simulink subsystem "PieroHFModel"  (R2023b)
settings: Solver=VariableStepAuto  StartTime=0.0  StopTime=10.0  RelTol=1e-3
settings Model: Creator=Hajar  LastModifiedBy=Hajar

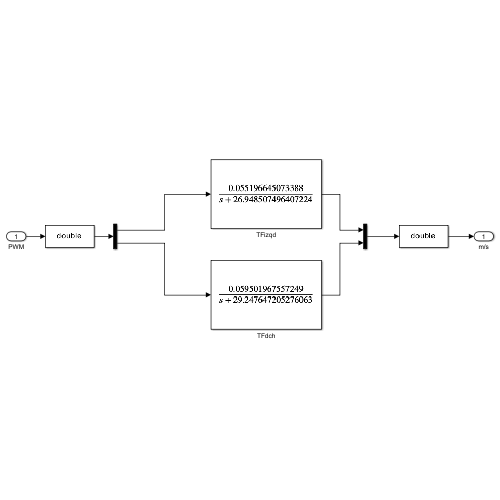
[thumbnail: Simulink's stored preview of the top-level diagram]
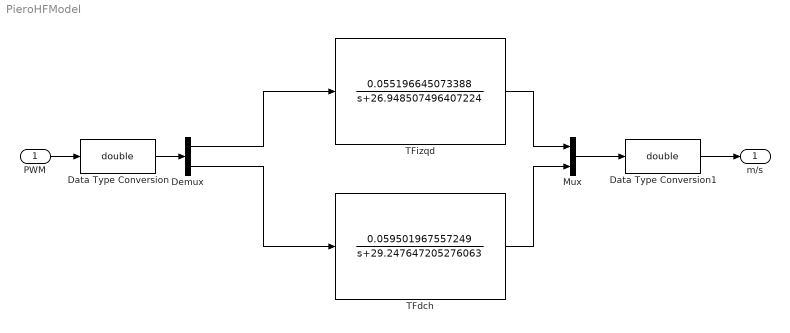
== system PieroHFModel ==
  PWM : Inport
  Data Type Conversion : DataTypeConversion  OutDataTypeStr=double  SaturateOnIntegerOverflow=off  RndMeth=Floor
  Data Type Conversion1 : DataTypeConversion  OutDataTypeStr=double  SaturateOnIntegerOverflow=off  RndMeth=Floor
  Demux : Demux  Outputs=2
  Mux : Mux  Inputs=2
  TFdch : TransferFcn  Numerator=0.059501967557249  Denominator=[1,29.247647205276063]
  TFizqd : TransferFcn  Numerator=0.055196645073388  Denominator=[1,26.948507496407224]
  m/s : Outport
  wires:
  Demux/1 -> TFizqd/1
  Demux/2 -> TFdch/1
  TFizqd/1 -> Mux/1
  TFdch/1 -> Mux/2
  PWM/1 -> Data Type Conversion/1
  Mux/1 -> Data Type Conversion1/1
  Data Type Conversion/1 -> Demux/1
  Data Type Conversion1/1 -> m/s/1
